simulink model "hybrid_new_eq_circuit_pascal5_single_shot_stack"  (R2019a)
settings: Solver=FixedStepAuto  StartTime=0.0  StopTime=sim_time  FixedStep=resolution  MinStep=0.001  RelTol=1e-4  EnableMultiTasking=on
values from neighbouring files (symbols this model uses):
  amps_in = double(amps_in)    [Sc.m]    (also in sc_model_single_shot_stack.m; test.m = 0; workspace_nedc_basic_sc.mat = 0; workspace_test_model.mat = 0)
  batt_c = [0.25 0.25 0.25 0.25 0.25 0.25 0.25]    [workspace_test_model.mat]
  batt_r = [1 1 1 1 1 1 1 1]    [workspace_test_model.mat]
  resolution = double(resolution)    [Sc.m]    (also in sc_model_single_shot.m = 0.1; sc_model_single_shot_stack.m = 0.1; workspace_test_model.mat = 10)
  tStep = resolution    (= 0.1)    [Sc.m]    (also in testHyb.m = 10; workspace_test_model.mat = 10)
undefined symbols (not defined in the file or in its folder): cCap, cR
libraries: powerlib x525, simulink x9
(part 2 of 8)

== system hybrid_new_eq_circuit_pascal5_single_shot_stack/Supercapacitor 2 ==
  note: 1x 4k
  note: 1x 550R
  note: 4x 625R
  note: 4x 1k4
  note: 6x 700R
  Bus Creator : BusCreator  Inputs=11
  Subsystem : Subsystem  mask{c=c(2), r_esr=r(2), r_leak=r_leak, v_init=v_init2}
      mask prompts: c "Capacitance /F"; r_esr "Series resistance /ohm"; r_leak "Leak resistance /ohm (inf for disabled)"; v_init "Initial capacitor voltage"
  Subsystem1 : Subsystem  mask{c=c(4), r_esr=r(4), r_leak=r_leak, v_init=v_init4}
      mask prompts: c "Capacitance /F"; r_esr "Series resistance /ohm"; r_leak "Leak resistance /ohm (inf for disabled)"; v_init "Initial capacitor voltage"
  Subsystem2 : Subsystem  mask{c=c(3), r_esr=r(3), r_leak=r_leak, v_init=v_init3}
      mask prompts: c "Capacitance /F"; r_esr "Series resistance /ohm"; r_leak "Leak resistance /ohm (inf for disabled)"; v_init "Initial capacitor voltage"
  Subsystem5 : Subsystem  mask{c=c(5), r_esr=r(5), r_leak=r_leak, v_init=v_init5}
      mask prompts: c "Capacitance /F"; r_esr "Series resistance /ohm"; r_leak "Leakage resistance /ohm (inf for disabled)"; v_init "Initial capacitor voltage"
  Subsystem8 : Subsystem  mask{c=c(1), r_esr=r(1), r_leak=r_leak, v_init=v_init1}
      mask prompts: c "Capacitance /F"; r_esr "Series resistance /ohm"; r_leak "Leakage resistance /ohm (inf for disabled)"; v_init "Initial capacitor voltage"
  v_cap_single : powerlib/Measurements/Voltage Measurement  PhasorSimulation=off  OutputType=Complex  PSBequivalent=0
      settings: SourceProductName=Simscape Electrical
  VCC_in : PMIOPort  Side=Left
  VSS_in : PMIOPort  Port=2  Side=Left
  VCC_out : PMIOPort  Port=3  Side=Right
  VSS_out : PMIOPort  Port=4  Side=Right
  v_r_out : Outport
  v_cap_out : Outport  Port=2
  i_leak_out : Outport  Port=3
  p_chg_out : Outport  Port=4
  p_leak_out : Outport  Port=5
  i_out : Outport  Port=6
  c_out : Outport  Port=7
  r_out : Outport  Port=8
  r_leak_out : Outport  Port=9
  bus_out : Outport  Port=10
  wires:
  Bus Creator/1 -> bus_out/1
  Subsystem5/10(l_out) -> Bus Creator/10
  v_cap_single/1 -> Bus Creator/11
  Subsystem2/7(Out7) -> Subsystem1/7(In7)
  Subsystem2/4(Out4) -> Subsystem1/4(In4)
  Subsystem2/3(Out3) -> Subsystem1/3(In3)
  Subsystem2/1(Out1) -> Subsystem1/1(In1)
  Subsystem2/9(Out9) -> Subsystem1/9(In9)
  Subsystem2/10(Out10) -> Subsystem1/10(In10)
  Subsystem2/2(Out2) -> Subsystem1/2(In2)
  Subsystem2/6(Out6) -> Subsystem1/6(In6)
  Subsystem2/8(Out8) -> Subsystem1/8(In8)
  Subsystem2/5(Out5) -> Subsystem1/5(In5)
  Subsystem/5(Out5) -> Subsystem2/5(In5)
  Subsystem/4(Out4) -> Subsystem2/4(In4)
  Subsystem/7(Out7) -> Subsystem2/7(In7)
  Subsystem/9(Out9) -> Subsystem2/9(In9)
  Subsystem/6(Out6) -> Subsystem2/6(In6)
  Subsystem/2(Out2) -> Subsystem2/2(In2)
  Subsystem/1(Out1) -> Subsystem2/1(In1)
  Subsystem/8(Out8) -> Subsystem2/8(In8)
  Subsystem/10(Out10) -> Subsystem2/10(In10)
  Subsystem/3(Out3) -> Subsystem2/3(In3)
  Subsystem1/1(Out1) -> Subsystem5/1(v_r_in)
  Subsystem1/2(Out2) -> Subsystem5/2(v_cap_in)
  Subsystem1/5(Out5) -> Subsystem5/5(p_leak_in)
  Subsystem1/10(Out10) -> Subsystem5/10(l_in)
  Subsystem1/3(Out3) -> Subsystem5/3(i_leak_in)
  Subsystem1/9(Out9) -> Subsystem5/9(r_leak_in)
  Subsystem1/7(Out7) -> Subsystem5/7(c_in)
  Subsystem1/4(Out4) -> Subsystem5/4(p_chg_in)
  Subsystem1/8(Out8) -> Subsystem5/8(r_in)
  Subsystem1/6(Out6) -> Subsystem5/6(i_in)
  Subsystem8/2(v_cap_out) -> Subsystem/2(In2)
  Subsystem8/1(v_r_out) -> Subsystem/1(In1)
  Subsystem8/7(c_out) -> Subsystem/7(In7)
  Subsystem8/5(p_leak_out) -> Subsystem/5(In5)
  Subsystem8/8(r_out) -> Subsystem/8(In8)
  Subsystem8/10(l_out) -> Subsystem/10(In10)
  Subsystem8/4(p_chg_out) -> Subsystem/4(In4)
  Subsystem8/9(r_leak_out) -> Subsystem/9(In9)
  Subsystem8/6(i_out) -> Subsystem/6(In6)
  Subsystem8/3(i_leak_out) -> Subsystem/3(In3)
  Subsystem5/1(v_r_out) -> v_r_out/1, Bus Creator/1
  Subsystem5/9(r_leak_out) -> r_leak_out/1, Bus Creator/9
  Subsystem5/2(v_cap_out) -> v_cap_out/1, Bus Creator/2
  Subsystem5/8(r_out) -> r_out/1, Bus Creator/8
  Subsystem5/3(i_leak_out) -> i_leak_out/1, Bus Creator/3
  Subsystem5/7(c_out) -> c_out/1, Bus Creator/7
  Subsystem5/4(p_chg_out) -> p_chg_out/1, Bus Creator/4
  Subsystem5/6(i_out) -> i_out/1, Bus Creator/6
  Subsystem5/5(p_leak_out) -> p_leak_out/1, Bus Creator/5
  connections:
  VSS_out/RConn1 -- v_cap_single/LConn2 -- Subsystem5/RConn2
  Subsystem5/RConn1 -- v_cap_single/LConn1 -- VCC_out/RConn1
  Subsystem1/LConn1 -- Subsystem2/RConn1
  Subsystem1/LConn2 -- Subsystem2/RConn2
  Subsystem/RConn2 -- Subsystem2/LConn2
  Subsystem/RConn1 -- Subsystem2/LConn1
  Subsystem1/RConn1 -- Subsystem5/LConn1
  Subsystem1/RConn2 -- Subsystem5/LConn2
  Subsystem8/RConn1 -- Subsystem/LConn1
  Subsystem8/RConn2 -- Subsystem/LConn2
  VSS_in/RConn1 -- Subsystem8/LConn2
  Subsystem8/LConn1 -- VCC_in/RConn1

== system hybrid_new_eq_circuit_pascal5_single_shot_stack/Supercapacitor 3 ==
  note: 6x 700R
  note: 4x 1k4
  note: 4x 625R
  note: 1x 550R
  note: 1x 4k
  Bus Creator : BusCreator  Inputs=11
  Subsystem : Subsystem  mask{c=c(2), r_esr=r(2), r_leak=r_leak, v_init=v_init2}
      mask prompts: c "Capacitance /F"; r_esr "Series resistance /ohm"; r_leak "Leak resistance /ohm (inf for disabled)"; v_init "Initial capacitor voltage"
  Subsystem1 : Subsystem  mask{c=c(4), r_esr=r(4), r_leak=r_leak, v_init=v_init4}
      mask prompts: c "Capacitance /F"; r_esr "Series resistance /ohm"; r_leak "Leak resistance /ohm (inf for disabled)"; v_init "Initial capacitor voltage"
  Subsystem2 : Subsystem  mask{c=c(3), r_esr=r(3), r_leak=r_leak, v_init=v_init3}
      mask prompts: c "Capacitance /F"; r_esr "Series resistance /ohm"; r_leak "Leak resistance /ohm (inf for disabled)"; v_init "Initial capacitor voltage"
  Subsystem5 : Subsystem  mask{c=c(5), r_esr=r(5), r_leak=r_leak, v_init=v_init5}
      mask prompts: c "Capacitance /F"; r_esr "Series resistance /ohm"; r_leak "Leakage resistance /ohm (inf for disabled)"; v_init "Initial capacitor voltage"
  Subsystem8 : Subsystem  mask{c=c(1), r_esr=r(1), r_leak=r_leak, v_init=v_init1}
      mask prompts: c "Capacitance /F"; r_esr "Series resistance /ohm"; r_leak "Leakage resistance /ohm (inf for disabled)"; v_init "Initial capacitor voltage"
  v_cap_single : powerlib/Measurements/Voltage Measurement  PhasorSimulation=off  OutputType=Complex  PSBequivalent=0
      settings: SourceProductName=Simscape Electrical
  VCC_in : PMIOPort  Side=Left
  VSS_in : PMIOPort  Port=2  Side=Left
  VCC_out : PMIOPort  Port=3  Side=Right
  VSS_out : PMIOPort  Port=4  Side=Right
  v_r_out : Outport
  v_cap_out : Outport  Port=2
  i_leak_out : Outport  Port=3
  p_chg_out : Outport  Port=4
  p_leak_out : Outport  Port=5
  i_out : Outport  Port=6
  c_out : Outport  Port=7
  r_out : Outport  Port=8
  r_leak_out : Outport  Port=9
  bus_out : Outport  Port=10
  wires:
  Subsystem5/5(p_leak_out) -> Bus Creator/5, p_leak_out/1
  Subsystem5/6(i_out) -> Bus Creator/6, i_out/1
  Subsystem5/4(p_chg_out) -> Bus Creator/4, p_chg_out/1
  Subsystem5/7(c_out) -> Bus Creator/7, c_out/1
  Subsystem5/3(i_leak_out) -> Bus Creator/3, i_leak_out/1
  Subsystem5/8(r_out) -> Bus Creator/8, r_out/1
  Subsystem5/2(v_cap_out) -> Bus Creator/2, v_cap_out/1
  Subsystem5/9(r_leak_out) -> Bus Creator/9, r_leak_out/1
  Subsystem5/1(v_r_out) -> Bus Creator/1, v_r_out/1
  Subsystem8/3(i_leak_out) -> Subsystem/3(In3)
  Subsystem8/6(i_out) -> Subsystem/6(In6)
  Subsystem8/9(r_leak_out) -> Subsystem/9(In9)
  Subsystem8/4(p_chg_out) -> Subsystem/4(In4)
  Subsystem8/10(l_out) -> Subsystem/10(In10)
  Subsystem8/8(r_out) -> Subsystem/8(In8)
  Subsystem8/5(p_leak_out) -> Subsystem/5(In5)
  Subsystem8/7(c_out) -> Subsystem/7(In7)
  Subsystem8/1(v_r_out) -> Subsystem/1(In1)
  Subsystem8/2(v_cap_out) -> Subsystem/2(In2)
  Subsystem1/6(Out6) -> Subsystem5/6(i_in)
  Subsystem1/8(Out8) -> Subsystem5/8(r_in)
  Subsystem1/4(Out4) -> Subsystem5/4(p_chg_in)
  Subsystem1/7(Out7) -> Subsystem5/7(c_in)
  Subsystem1/9(Out9) -> Subsystem5/9(r_leak_in)
  Subsystem1/3(Out3) -> Subsystem5/3(i_leak_in)
  Subsystem1/10(Out10) -> Subsystem5/10(l_in)
  Subsystem1/5(Out5) -> Subsystem5/5(p_leak_in)
  Subsystem1/2(Out2) -> Subsystem5/2(v_cap_in)
  Subsystem1/1(Out1) -> Subsystem5/1(v_r_in)
  Subsystem/3(Out3) -> Subsystem2/3(In3)
  Subsystem/10(Out10) -> Subsystem2/10(In10)
  Subsystem/8(Out8) -> Subsystem2/8(In8)
  Subsystem/1(Out1) -> Subsystem2/1(In1)
  Subsystem/2(Out2) -> Subsystem2/2(In2)
  Subsystem/6(Out6) -> Subsystem2/6(In6)
  Subsystem/9(Out9) -> Subsystem2/9(In9)
  Subsystem/7(Out7) -> Subsystem2/7(In7)
  Subsystem/4(Out4) -> Subsystem2/4(In4)
  Subsystem/5(Out5) -> Subsystem2/5(In5)
  Subsystem2/5(Out5) -> Subsystem1/5(In5)
  Subsystem2/8(Out8) -> Subsystem1/8(In8)
  Subsystem2/6(Out6) -> Subsystem1/6(In6)
  Subsystem2/2(Out2) -> Subsystem1/2(In2)
  Subsystem2/10(Out10) -> Subsystem1/10(In10)
  Subsystem2/9(Out9) -> Subsystem1/9(In9)
  Subsystem2/1(Out1) -> Subsystem1/1(In1)
  Subsystem2/3(Out3) -> Subsystem1/3(In3)
  Subsystem2/4(Out4) -> Subsystem1/4(In4)
  Subsystem2/7(Out7) -> Subsystem1/7(In7)
  v_cap_single/1 -> Bus Creator/11
  Subsystem5/10(l_out) -> Bus Creator/10
  Bus Creator/1 -> bus_out/1
  connections:
  Subsystem8/LConn1 -- VCC_in/RConn1
  VSS_in/RConn1 -- Subsystem8/LConn2
  Subsystem8/RConn2 -- Subsystem/LConn2
  Subsystem8/RConn1 -- Subsystem/LConn1
  Subsystem1/RConn2 -- Subsystem5/LConn2
  Subsystem1/RConn1 -- Subsystem5/LConn1
  Subsystem/RConn1 -- Subsystem2/LConn1
  Subsystem/RConn2 -- Subsystem2/LConn2
  Subsystem1/LConn2 -- Subsystem2/RConn2
  Subsystem1/LConn1 -- Subsystem2/RConn1
  VCC_out/RConn1 -- v_cap_single/LConn1 -- Subsystem5/RConn1
  Subsystem5/RConn2 -- v_cap_single/LConn2 -- VSS_out/RConn1

== system hybrid_new_eq_circuit_pascal5_single_shot_stack/Battery 1/Subsystem ==
  In1 : Inport
  In2 : Inport  Port=2
  In3 : Inport  Port=3
  In4 : Inport  Port=4
  In5 : Inport  Port=5
  In6 : Inport  Port=6
  In7 : Inport  Port=7
  In8 : Inport  Port=8
  In9 : Inport  Port=9
  In10 : Inport  Port=10
  Subsystem1 : Subsystem  mask{c=c(5), r_esr=r(5), r_leak=r_leak, v_init=v_init(5)}
      mask prompts: c "Capacitance /F"; r_esr "Series resistance /ohm"; r_leak "Leakage resistance /ohm (inf for disabled)"; v_init "Initial capacitor voltage"
  Subsystem2 : Subsystem  mask{c=c(6), r_esr=r(6), r_leak=r_leak, v_init=v_init(6)}
      mask prompts: c "Capacitance /F"; r_esr "Series resistance /ohm"; r_leak "Leakage resistance /ohm (inf for disabled)"; v_init "Initial capacitor voltage"
  Subsystem3 : Subsystem  mask{c=c(7), r_esr=r(7), r_leak=r_leak, v_init=v_init(7)}
      mask prompts: c "Capacitance /F"; r_esr "Series resistance /ohm"; r_leak "Leakage resistance /ohm (inf for disabled)"; v_init "Initial capacitor voltage"
  Subsystem5 : Subsystem  mask{c=c(4), r_esr=r(4), r_leak=r_leak, v_init=v_init(4)}
      mask prompts: c "Capacitance /F"; r_esr "Series resistance /ohm"; r_leak "Leakage resistance /ohm (inf for disabled)"; v_init "Initial capacitor voltage"
  VCC_in : PMIOPort  Side=Left
  VCC_out : PMIOPort  Port=2  Side=Right
  VSS_in : PMIOPort  Port=3  Side=Left
  VSS_out : PMIOPort  Port=4  Side=Right
  Out1 : Outport
  Out2 : Outport  Port=2
  Out3 : Outport  Port=3
  Out4 : Outport  Port=4
  Out5 : Outport  Port=5
  Out6 : Outport  Port=6
  Out7 : Outport  Port=7
  Out8 : Outport  Port=8
  Out9 : Outport  Port=9
  Out10 : Outport  Port=10
  wires:
  In2/1 -> Subsystem5/2(v_cap_in)
  In9/1 -> Subsystem5/9(r_leak_in)
  In6/1 -> Subsystem5/6(i_in)
  In5/1 -> Subsystem5/5(p_leak_in)
  In4/1 -> Subsystem5/4(p_chg_in)
  In7/1 -> Subsystem5/7(c_in)
  In1/1 -> Subsystem5/1(v_r_in)
  In10/1 -> Subsystem5/10(l_in)
  In3/1 -> Subsystem5/3(i_leak_in)
  In8/1 -> Subsystem5/8(r_in)
  Subsystem5/1(v_r_out) -> Subsystem1/1(v_r_in)
  Subsystem5/2(v_cap_out) -> Subsystem1/2(v_cap_in)
  Subsystem5/3(i_leak_out) -> Subsystem1/3(i_leak_in)
  Subsystem5/4(p_chg_out) -> Subsystem1/4(p_chg_in)
  Subsystem5/5(p_leak_out) -> Subsystem1/5(p_leak_in)
  Subsystem5/6(i_out) -> Subsystem1/6(i_in)
  Subsystem5/7(c_out) -> Subsystem1/7(c_in)
  Subsystem5/8(r_out) -> Subsystem1/8(r_in)
  Subsystem5/9(r_leak_out) -> Subsystem1/9(r_leak_in)
  Subsystem5/10(l_out) -> Subsystem1/10(l_in)
  Subsystem1/1(v_r_out) -> Subsystem2/1(v_r_in)
  Subsystem1/2(v_cap_out) -> Subsystem2/2(v_cap_in)
  Subsystem1/3(i_leak_out) -> Subsystem2/3(i_leak_in)
  Subsystem1/4(p_chg_out) -> Subsystem2/4(p_chg_in)
  Subsystem1/5(p_leak_out) -> Subsystem2/5(p_leak_in)
  Subsystem1/6(i_out) -> Subsystem2/6(i_in)
  Subsystem1/7(c_out) -> Subsystem2/7(c_in)
  Subsystem1/8(r_out) -> Subsystem2/8(r_in)
  Subsystem1/9(r_leak_out) -> Subsystem2/9(r_leak_in)
  Subsystem1/10(l_out) -> Subsystem2/10(l_in)
  Subsystem2/1(v_r_out) -> Subsystem3/1(v_r_in)
  Subsystem2/2(v_cap_out) -> Subsystem3/2(v_cap_in)
  Subsystem2/3(i_leak_out) -> Subsystem3/3(i_leak_in)
  Subsystem2/4(p_chg_out) -> Subsystem3/4(p_chg_in)
  Subsystem2/5(p_leak_out) -> Subsystem3/5(p_leak_in)
  Subsystem2/6(i_out) -> Subsystem3/6(i_in)
  Subsystem2/7(c_out) -> Subsystem3/7(c_in)
  Subsystem2/8(r_out) -> Subsystem3/8(r_in)
  Subsystem2/9(r_leak_out) -> Subsystem3/9(r_leak_in)
  Subsystem2/10(l_out) -> Subsystem3/10(l_in)
  Subsystem3/1(v_r_out) -> Out1/1
  Subsystem3/2(v_cap_out) -> Out2/1
  Subsystem3/3(i_leak_out) -> Out3/1
  Subsystem3/4(p_chg_out) -> Out4/1
  Subsystem3/5(p_leak_out) -> Out5/1
  Subsystem3/6(i_out) -> Out6/1
  Subsystem3/7(c_out) -> Out7/1
  Subsystem3/8(r_out) -> Out8/1
  Subsystem3/9(r_leak_out) -> Out9/1
  Subsystem3/10(l_out) -> Out10/1
  connections:
  Subsystem5/LConn1 -- VCC_in/RConn1
  Subsystem5/LConn2 -- VSS_in/RConn1
  Subsystem5/RConn1 -- Subsystem1/LConn1
  Subsystem5/RConn2 -- Subsystem1/LConn2
  Subsystem1/RConn1 -- Subsystem2/LConn1
  Subsystem1/RConn2 -- Subsystem2/LConn2
  Subsystem2/RConn1 -- Subsystem3/LConn1
  Subsystem2/RConn2 -- Subsystem3/LConn2
  Subsystem3/RConn1 -- VCC_out/RConn1
  Subsystem3/RConn2 -- VSS_out/RConn1

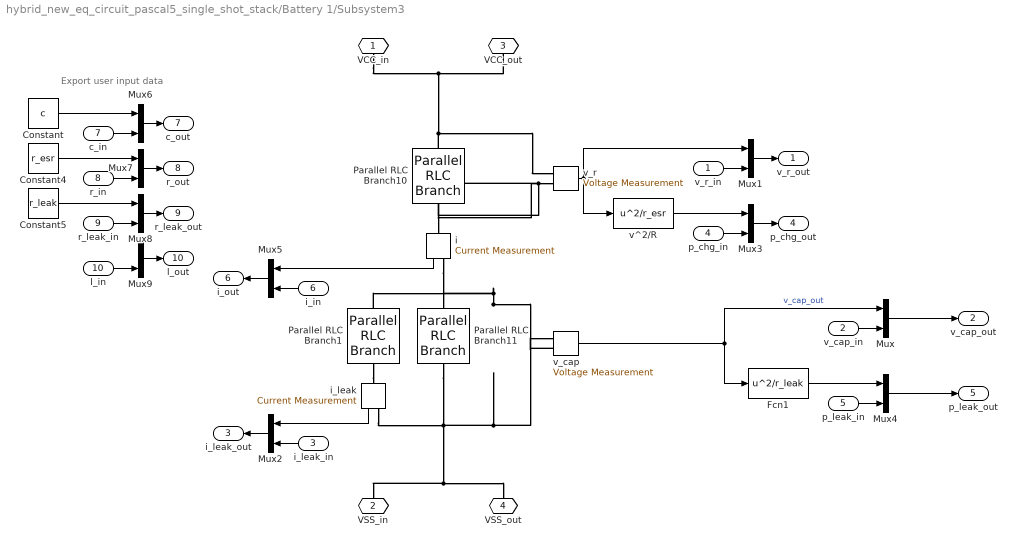
== system hybrid_new_eq_circuit_pascal5_single_shot_stack/Battery 1/Subsystem3 ==
  note: Export user input data
  v_r_in : Inport
  v_cap_in : Inport  Port=2
  i_leak_in : Inport  Port=3
  p_chg_in : Inport  Port=4
  p_leak_in : Inport  Port=5
  i_in : Inport  Port=6
  c_in : Inport  Port=7
  r_in : Inport  Port=8
  r_leak_in : Inport  Port=9
  l_in : Inport  Port=10
  Constant : Constant  Value=c
  Constant4 : Constant  Value=r_esr
  Constant5 : Constant  Value=r_leak
  Fcn1 : Fcn  Expr=u^2/r_leak
  Mux{,1..9} (10 alike) : Mux  Inputs=2
  Parallel RLC Branch1 : powerlib/Elements/Parallel RLC Branch  LConnTagsString=a  RConnTagsString=__new0  BranchType=R  Resistance=r_esr  Inductance=1e-3  SetiL0=off  InitialCurrent=0  Capacitance=1e-6  Setx0=off  InitialVoltage=0  Measurements=None
      settings: SourceProductName=Simscape Electrical
  Parallel RLC Branch10 : powerlib/Elements/Parallel RLC Branch  LConnTagsString=a  RConnTagsString=__new0  BranchType=R  Resistance=0.000001  Inductance=1e-3  SetiL0=off  InitialCurrent=0  Capacitance=1e-6  Setx0=off  InitialVoltage=0  Measurements=None
      settings: SourceProductName=Simscape Electrical
  Parallel RLC Branch11 : powerlib/Elements/Parallel RLC Branch  LConnTagsString=a  RConnTagsString=__new0  BranchType=C  Resistance=1  Inductance=1e-3  SetiL0=off  InitialCurrent=0  Capacitance=c  Setx0=on  InitialVoltage=v_init  Measurements=None
      settings: SourceProductName=Simscape Electrical
  i : powerlib/Measurements/Current Measurement  PhasorSimulation=off  OutputType=Complex  PSBequivalent=0
      settings: SourceProductName=Simscape Electrical
  i_leak : powerlib/Measurements/Current Measurement  PhasorSimulation=off  OutputType=Complex  PSBequivalent=0
      settings: SourceProductName=Simscape Electrical
  v^2/R : Fcn  Expr=u^2/r_esr
  v_cap : powerlib/Measurements/Voltage Measurement  PhasorSimulation=off  OutputType=Magnitude  PSBequivalent=0
      settings: SourceProductName=Simscape Electrical
  v_r : powerlib/Measurements/Voltage Measurement  PhasorSimulation=off  OutputType=Complex  PSBequivalent=0
      settings: SourceProductName=Simscape Electrical
  VCC_in : PMIOPort  Side=Left
  VSS_in : PMIOPort  Port=2  Side=Left
  VCC_out : PMIOPort  Tag=PMCPort  Port=3  Side=Right
  VSS_out : PMIOPort  Tag=PMCPort  Port=4  Side=Right
  v_r_out : Outport
  v_cap_out : Outport  Port=2
  i_leak_out : Outport  Port=3
  p_chg_out : Outport  Port=4
  p_leak_out : Outport  Port=5
  i_out : Outport  Port=6
  c_out : Outport  Port=7
  r_out : Outport  Port=8
  r_leak_out : Outport  Port=9
  l_out : Outport  Port=10
  wires:
  i_leak/1 -> Mux2/1
  v_r/1 -> Mux1/1, v^2/R/1
  Mux6/1 -> c_out/1
  Mux7/1 -> r_out/1
  Mux8/1 -> r_leak_out/1
  Mux9/1 -> l_out/1
  Constant/1 -> Mux6/1
  Constant4/1 -> Mux7/1
  Constant5/1 -> Mux8/1
  ? -> Mux9/1
  c_in/1 -> Mux6/2
  l_in/1 -> Mux9/2
  r_leak_in/1 -> Mux8/2
  r_in/1 -> Mux7/2
  p_chg_in/1 -> Mux3/2
  Mux3/1 -> p_chg_out/1
  v_r_in/1 -> Mux1/2
  Mux1/1 -> v_r_out/1
  v^2/R/1 -> Mux3/1
  Mux2/1 -> i_leak_out/1
  i_leak_in/1 -> Mux2/2
  i/1 -> Mux5/1
  Mux5/1 -> i_out/1
  i_in/1 -> Mux5/2
  p_leak_in/1 -> Mux4/2
  Mux4/1 -> p_leak_out/1
  Mux/1 -> v_cap_out/1
  v_cap_in/1 -> Mux/2
  Fcn1/1 -> Mux4/1
  v_cap/1 -> Fcn1/1, Mux/1  "v_cap_out"
  connections:
  VCC_in/RConn1 -- VCC_out/RConn1 -- v_r/LConn1 -- Parallel RLC Branch10/LConn1
  Parallel RLC Branch1/RConn1 -- i_leak/LConn1
  VSS_out/RConn1 -- VSS_in/RConn1 -- i_leak/RConn1 -- Parallel RLC Branch11/RConn1 -- v_cap/LConn2
  Parallel RLC Branch1/LConn1 -- i/RConn1 -- Parallel RLC Branch11/LConn1 -- v_cap/LConn1
  v_r/LConn2 -- Parallel RLC Branch10/RConn1 -- i/LConn1

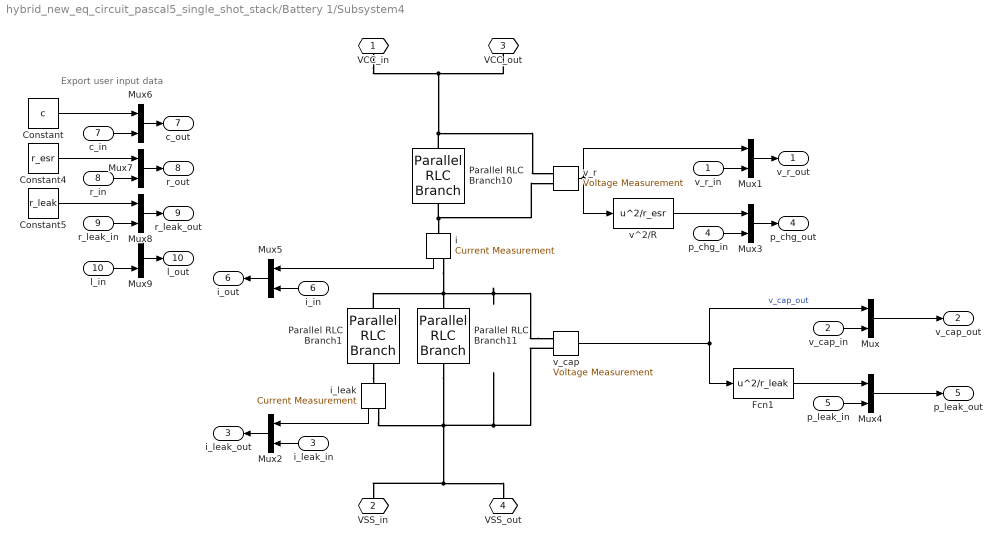
== system hybrid_new_eq_circuit_pascal5_single_shot_stack/Battery 1/Subsystem4 ==
  note: Export user input data
  v_r_in : Inport
  v_cap_in : Inport  Port=2
  i_leak_in : Inport  Port=3
  p_chg_in : Inport  Port=4
  p_leak_in : Inport  Port=5
  i_in : Inport  Port=6
  c_in : Inport  Port=7
  r_in : Inport  Port=8
  r_leak_in : Inport  Port=9
  l_in : Inport  Port=10
  Constant : Constant  Value=c
  Constant4 : Constant  Value=r_esr
  Constant5 : Constant  Value=r_leak
  Fcn1 : Fcn  Expr=u^2/r_leak
  Mux{,1..9} (10 alike) : Mux  Inputs=2
  Parallel RLC Branch1 : powerlib/Elements/Parallel RLC Branch  LConnTagsString=a  RConnTagsString=__new0  BranchType=R  Resistance=r_esr  Inductance=1e-3  SetiL0=off  InitialCurrent=0  Capacitance=1e-6  Setx0=off  InitialVoltage=0  Measurements=None
      settings: SourceProductName=Simscape Electrical
  Parallel RLC Branch10 : powerlib/Elements/Parallel RLC Branch  LConnTagsString=a  RConnTagsString=__new0  BranchType=R  Resistance=0.000001  Inductance=1e-3  SetiL0=off  InitialCurrent=0  Capacitance=1e-6  Setx0=off  InitialVoltage=0  Measurements=None
      settings: SourceProductName=Simscape Electrical
  Parallel RLC Branch11 : powerlib/Elements/Parallel RLC Branch  LConnTagsString=a  RConnTagsString=__new0  BranchType=C  Resistance=1  Inductance=1e-3  SetiL0=off  InitialCurrent=0  Capacitance=c  Setx0=on  InitialVoltage=v_init  Measurements=None
      settings: SourceProductName=Simscape Electrical
  i : powerlib/Measurements/Current Measurement  PhasorSimulation=off  OutputType=Complex  PSBequivalent=0
      settings: SourceProductName=Simscape Electrical
  i_leak : powerlib/Measurements/Current Measurement  PhasorSimulation=off  OutputType=Complex  PSBequivalent=0
      settings: SourceProductName=Simscape Electrical
  v^2/R : Fcn  Expr=u^2/r_esr
  v_cap : powerlib/Measurements/Voltage Measurement  PhasorSimulation=off  OutputType=Magnitude  PSBequivalent=0
      settings: SourceProductName=Simscape Electrical
  v_r : powerlib/Measurements/Voltage Measurement  PhasorSimulation=off  OutputType=Complex  PSBequivalent=0
      settings: SourceProductName=Simscape Electrical
  VCC_in : PMIOPort  Side=Left
  VSS_in : PMIOPort  Port=2  Side=Left
  VCC_out : PMIOPort  Tag=PMCPort  Port=3  Side=Right
  VSS_out : PMIOPort  Tag=PMCPort  Port=4  Side=Right
  v_r_out : Outport
  v_cap_out : Outport  Port=2
  i_leak_out : Outport  Port=3
  p_chg_out : Outport  Port=4
  p_leak_out : Outport  Port=5
  i_out : Outport  Port=6
  c_out : Outport  Port=7
  r_out : Outport  Port=8
  r_leak_out : Outport  Port=9
  l_out : Outport  Port=10
  wires:
  Fcn1/1 -> Mux4/1
  v_cap_in/1 -> Mux/2
  Mux/1 -> v_cap_out/1
  Mux4/1 -> p_leak_out/1
  p_leak_in/1 -> Mux4/2
  i_in/1 -> Mux5/2
  Mux5/1 -> i_out/1
  i/1 -> Mux5/1
  i_leak_in/1 -> Mux2/2
  Mux2/1 -> i_leak_out/1
  v^2/R/1 -> Mux3/1
  Mux1/1 -> v_r_out/1
  v_r_in/1 -> Mux1/2
  Mux3/1 -> p_chg_out/1
  p_chg_in/1 -> Mux3/2
  r_in/1 -> Mux7/2
  r_leak_in/1 -> Mux8/2
  l_in/1 -> Mux9/2
  c_in/1 -> Mux6/2
  ? -> Mux9/1
  Constant5/1 -> Mux8/1
  Constant4/1 -> Mux7/1
  Constant/1 -> Mux6/1
  Mux9/1 -> l_out/1
  Mux8/1 -> r_leak_out/1
  Mux7/1 -> r_out/1
  Mux6/1 -> c_out/1
  v_r/1 -> v^2/R/1, Mux1/1
  i_leak/1 -> Mux2/1
  v_cap/1 -> Mux/1, Fcn1/1  "v_cap_out"
  connections:
  i/LConn1 -- Parallel RLC Branch10/RConn1 -- v_r/LConn2
  Parallel RLC Branch10/LConn1 -- VCC_in/RConn1 -- VCC_out/RConn1 -- v_r/LConn1
  v_cap/LConn1 -- Parallel RLC Branch11/LConn1 -- i/RConn1 -- Parallel RLC Branch1/LConn1
  v_cap/LConn2 -- Parallel RLC Branch11/RConn1 -- i_leak/RConn1 -- VSS_in/RConn1 -- VSS_out/RConn1
  Parallel RLC Branch1/RConn1 -- i_leak/LConn1

== system hybrid_new_eq_circuit_pascal5_single_shot_stack/Battery 1/Subsystem8 ==
  note: Export user input data
  Constant : Constant  Value=c
  Constant4 : Constant  Value=r_esr
  Constant5 : Constant  Value=r_leak
  Fcn1 : Fcn  Expr=u^2/r_leak
  Parallel RLC Branch1 : powerlib/Elements/Parallel RLC Branch  LConnTagsString=a  RConnTagsString=__new0  BranchType=R  Resistance=r_leak  Inductance=1e-3  SetiL0=off  InitialCurrent=0  Capacitance=1e-6  Setx0=off  InitialVoltage=0  Measurements=None
      settings: SourceProductName=Simscape Electrical
  Parallel RLC Branch10 : powerlib/Elements/Parallel RLC Branch  LConnTagsString=a  RConnTagsString=__new0  BranchType=R  Resistance=0.000001  Inductance=1e-3  SetiL0=off  InitialCurrent=0  Capacitance=1e-6  Setx0=off  InitialVoltage=0  Measurements=None
      settings: SourceProductName=Simscape Electrical
  Parallel RLC Branch11 : powerlib/Elements/Parallel RLC Branch  LConnTagsString=a  RConnTagsString=__new0  BranchType=C  Resistance=1  Inductance=1e-3  SetiL0=off  InitialCurrent=0  Capacitance=c  Setx0=on  InitialVoltage=v_init  Measurements=None
      settings: SourceProductName=Simscape Electrical
  i : powerlib/Measurements/Current Measurement  PhasorSimulation=off  OutputType=Complex  PSBequivalent=0
      settings: SourceProductName=Simscape Electrical
  i_leak : powerlib/Measurements/Current Measurement  PhasorSimulation=off  OutputType=Complex  PSBequivalent=0
      settings: SourceProductName=Simscape Electrical
  v^2/R : Fcn  Expr=u^2/r_esr
  v_cap : powerlib/Measurements/Voltage Measurement  PhasorSimulation=off  OutputType=Magnitude  PSBequivalent=0
      settings: SourceProductName=Simscape Electrical
  v_r : powerlib/Measurements/Voltage Measurement  PhasorSimulation=off  OutputType=Complex  PSBequivalent=0
      settings: SourceProductName=Simscape Electrical
  VCC_in : PMIOPort  Side=Left
  VSS_in : PMIOPort  Port=2  Side=Left
  VCC_out : PMIOPort  Tag=PMCPort  Port=3  Side=Right
  VSS_out : PMIOPort  Tag=PMCPort  Port=4  Side=Right
  v_r_out : Outport
  v_cap_out : Outport  Port=2
  i_leak_out : Outport  Port=3
  p_chg_out : Outport  Port=4
  p_leak_out : Outport  Port=5
  i_out : Outport  Port=6
  c_out : Outport  Port=7
  r_out : Outport  Port=8
  r_leak_out : Outport  Port=9
  l_out : Outport  Port=10
  wires:
  v^2/R/1 -> p_chg_out/1
  Fcn1/1 -> p_leak_out/1
  v_cap/1 -> Fcn1/1, v_cap_out/1  "v_cap_out"
  i/1 -> i_out/1
  ? -> l_out/1
  Constant5/1 -> r_leak_out/1
  Constant4/1 -> r_out/1
  Constant/1 -> c_out/1
  v_r/1 -> v^2/R/1, v_r_out/1
  i_leak/1 -> i_leak_out/1
  connections:
  v_r/LConn2 -- Parallel RLC Branch10/RConn1 -- i/LConn1
  Parallel RLC Branch1/RConn1 -- i_leak/LConn1
  Parallel RLC Branch10/LConn1 -- v_r/LConn1 -- VCC_out/RConn1 -- VCC_in/RConn1
  v_cap/LConn1 -- i/RConn1 -- Parallel RLC Branch1/LConn1 -- Parallel RLC Branch11/LConn1
  VSS_in/RConn1 -- VSS_out/RConn1 -- i_leak/RConn1 -- v_cap/LConn2 -- Parallel RLC Branch11/RConn1

== system hybrid_new_eq_circuit_pascal5_single_shot_stack/Battery 2/Bus Merge2 ==
  bus_1_in : Inport
  bus_2_in : Inport  Port=2
  Bus Creator : BusCreator  Inputs=11
  Bus Selector : BusSelector  OutputSignals=signal1,v_cap_out,signal3,signal4,signal5,signal6,signal7,signal8,signal9,signal10,signal11
  Bus Selector1 : BusSelector  OutputSignals=signal1,v_cap_out,signal3,signal4,signal5,signal6,signal7,signal8,signal9,signal10,signal11
  Mux{1..11} (11 alike) : Mux  Inputs=2
  bus_out : Outport
  wires:
  bus_1_in/1 -> Bus Selector/1
  bus_2_in/1 -> Bus Selector1/1
  Bus Creator/1 -> bus_out/1
  Bus Selector/1 -> Mux1/1  "<signal1>"
  Bus Selector1/2 -> Mux2/2  "<v_cap_out>"
  Bus Selector/3 -> Mux3/1  "<signal3>"
  Bus Selector1/4 -> Mux4/2  "<signal4>"
  Bus Selector/5 -> Mux5/1  "<signal5>"
  Bus Selector1/6 -> Mux6/1  "<signal6>"
  Bus Selector/7 -> Mux7/1  "<signal7>"
  Bus Selector1/8 -> Mux8/1  "<signal8>"
  Bus Selector1/10 -> Mux10/1  "<signal10>"
  Bus Selector/11 -> Mux11/1  "<signal11>"
  Bus Selector/9 -> Mux9/1  "<signal9>"
  Bus Selector/2 -> Mux2/1  "<v_cap_out>"
  Bus Selector/4 -> Mux4/1  "<signal4>"
  Bus Selector/6 -> Mux6/2  "<signal6>"
  Bus Selector/8 -> Mux8/2  "<signal8>"
  Bus Selector/10 -> Mux10/2  "<signal10>"
  Bus Selector1/1 -> Mux1/2  "<signal1>"
  Bus Selector1/3 -> Mux3/2  "<signal3>"
  Bus Selector1/5 -> Mux5/2  "<signal5>"
  Bus Selector1/7 -> Mux7/2  "<signal7>"
  Bus Selector1/9 -> Mux9/2  "<signal9>"
  Bus Selector1/11 -> Mux11/2  "<signal11>"
  Mux1/1 -> Bus Creator/1
  Mux3/1 -> Bus Creator/3
  Mux5/1 -> Bus Creator/5
  Mux7/1 -> Bus Creator/7
  Mux9/1 -> Bus Creator/9
  Mux11/1 -> Bus Creator/11
  Mux2/1 -> Bus Creator/2  "v_cap_out"
  Mux4/1 -> Bus Creator/4
  Mux6/1 -> Bus Creator/6
  Mux8/1 -> Bus Creator/8
  Mux10/1 -> Bus Creator/10

== system hybrid_new_eq_circuit_pascal5_single_shot_stack/Battery 2/Subsystem ==
  In1 : Inport
  In2 : Inport  Port=2
  In3 : Inport  Port=3
  In4 : Inport  Port=4
  In5 : Inport  Port=5
  In6 : Inport  Port=6
  In7 : Inport  Port=7
  In8 : Inport  Port=8
  In9 : Inport  Port=9
  In10 : Inport  Port=10
  Subsystem1 : Subsystem  mask{c=c(5), r_esr=r(5), r_leak=r_leak, v_init=v_init(5)}
      mask prompts: c "Capacitance /F"; r_esr "Series resistance /ohm"; r_leak "Leakage resistance /ohm (inf for disabled)"; v_init "Initial capacitor voltage"
  Subsystem2 : Subsystem  mask{c=c(6), r_esr=r(6), r_leak=r_leak, v_init=v_init(6)}
      mask prompts: c "Capacitance /F"; r_esr "Series resistance /ohm"; r_leak "Leakage resistance /ohm (inf for disabled)"; v_init "Initial capacitor voltage"
  Subsystem3 : Subsystem  mask{c=c(7), r_esr=r(7), r_leak=r_leak, v_init=v_init(7)}
      mask prompts: c "Capacitance /F"; r_esr "Series resistance /ohm"; r_leak "Leakage resistance /ohm (inf for disabled)"; v_init "Initial capacitor voltage"
  Subsystem5 : Subsystem  mask{c=c(4), r_esr=r(4), r_leak=r_leak, v_init=v_init(4)}
      mask prompts: c "Capacitance /F"; r_esr "Series resistance /ohm"; r_leak "Leakage resistance /ohm (inf for disabled)"; v_init "Initial capacitor voltage"
  Conn1 : PMIOPort  Side=Left
  Conn2 : PMIOPort  Port=2  Side=Right
  Conn3 : PMIOPort  Port=3  Side=Left
  Conn4 : PMIOPort  Port=4  Side=Right
  Out1 : Outport
  Out2 : Outport  Port=2
  Out3 : Outport  Port=3
  Out4 : Outport  Port=4
  Out5 : Outport  Port=5
  Out6 : Outport  Port=6
  Out7 : Outport  Port=7
  Out8 : Outport  Port=8
  Out9 : Outport  Port=9
  Out10 : Outport  Port=10
  wires:
  In2/1 -> Subsystem5/2(v_cap_in)
  In9/1 -> Subsystem5/9(r_leak_in)
  In6/1 -> Subsystem5/6(i_in)
  In5/1 -> Subsystem5/5(p_leak_in)
  In4/1 -> Subsystem5/4(p_chg_in)
  In7/1 -> Subsystem5/7(c_in)
  In1/1 -> Subsystem5/1(v_r_in)
  In10/1 -> Subsystem5/10(l_in)
  In3/1 -> Subsystem5/3(i_leak_in)
  In8/1 -> Subsystem5/8(r_in)
  Subsystem5/1(v_r_out) -> Subsystem1/1(v_r_in)
  Subsystem5/2(v_cap_out) -> Subsystem1/2(v_cap_in)
  Subsystem5/3(i_leak_out) -> Subsystem1/3(i_leak_in)
  Subsystem5/4(p_chg_out) -> Subsystem1/4(p_chg_in)
  Subsystem5/5(p_leak_out) -> Subsystem1/5(p_leak_in)
  Subsystem5/6(i_out) -> Subsystem1/6(i_in)
  Subsystem5/7(c_out) -> Subsystem1/7(c_in)
  Subsystem5/8(r_out) -> Subsystem1/8(r_in)
  Subsystem5/9(r_leak_out) -> Subsystem1/9(r_leak_in)
  Subsystem5/10(l_out) -> Subsystem1/10(l_in)
  Subsystem1/1(v_r_out) -> Subsystem2/1(v_r_in)
  Subsystem1/2(v_cap_out) -> Subsystem2/2(v_cap_in)
  Subsystem1/3(i_leak_out) -> Subsystem2/3(i_leak_in)
  Subsystem1/4(p_chg_out) -> Subsystem2/4(p_chg_in)
  Subsystem1/5(p_leak_out) -> Subsystem2/5(p_leak_in)
  Subsystem1/6(i_out) -> Subsystem2/6(i_in)
  Subsystem1/7(c_out) -> Subsystem2/7(c_in)
  Subsystem1/8(r_out) -> Subsystem2/8(r_in)
  Subsystem1/9(r_leak_out) -> Subsystem2/9(r_leak_in)
  Subsystem1/10(l_out) -> Subsystem2/10(l_in)
  Subsystem2/1(v_r_out) -> Subsystem3/1(v_r_in)
  Subsystem2/2(v_cap_out) -> Subsystem3/2(v_cap_in)
  Subsystem2/3(i_leak_out) -> Subsystem3/3(i_leak_in)
  Subsystem2/4(p_chg_out) -> Subsystem3/4(p_chg_in)
  Subsystem2/5(p_leak_out) -> Subsystem3/5(p_leak_in)
  Subsystem2/6(i_out) -> Subsystem3/6(i_in)
  Subsystem2/7(c_out) -> Subsystem3/7(c_in)
  Subsystem2/8(r_out) -> Subsystem3/8(r_in)
  Subsystem2/9(r_leak_out) -> Subsystem3/9(r_leak_in)
  Subsystem2/10(l_out) -> Subsystem3/10(l_in)
  Subsystem3/1(v_r_out) -> Out1/1
  Subsystem3/2(v_cap_out) -> Out2/1
  Subsystem3/3(i_leak_out) -> Out3/1
  Subsystem3/4(p_chg_out) -> Out4/1
  Subsystem3/5(p_leak_out) -> Out5/1
  Subsystem3/6(i_out) -> Out6/1
  Subsystem3/7(c_out) -> Out7/1
  Subsystem3/8(r_out) -> Out8/1
  Subsystem3/9(r_leak_out) -> Out9/1
  Subsystem3/10(l_out) -> Out10/1
  connections:
  Subsystem5/LConn1 -- Conn1/RConn1
  Subsystem5/LConn2 -- Conn3/RConn1
  Subsystem5/RConn1 -- Subsystem1/LConn1
  Subsystem5/RConn2 -- Subsystem1/LConn2
  Subsystem1/RConn1 -- Subsystem2/LConn1
  Subsystem1/RConn2 -- Subsystem2/LConn2
  Subsystem2/RConn1 -- Subsystem3/LConn1
  Subsystem2/RConn2 -- Subsystem3/LConn2
  Subsystem3/RConn1 -- Conn2/RConn1
  Subsystem3/RConn2 -- Conn4/RConn1

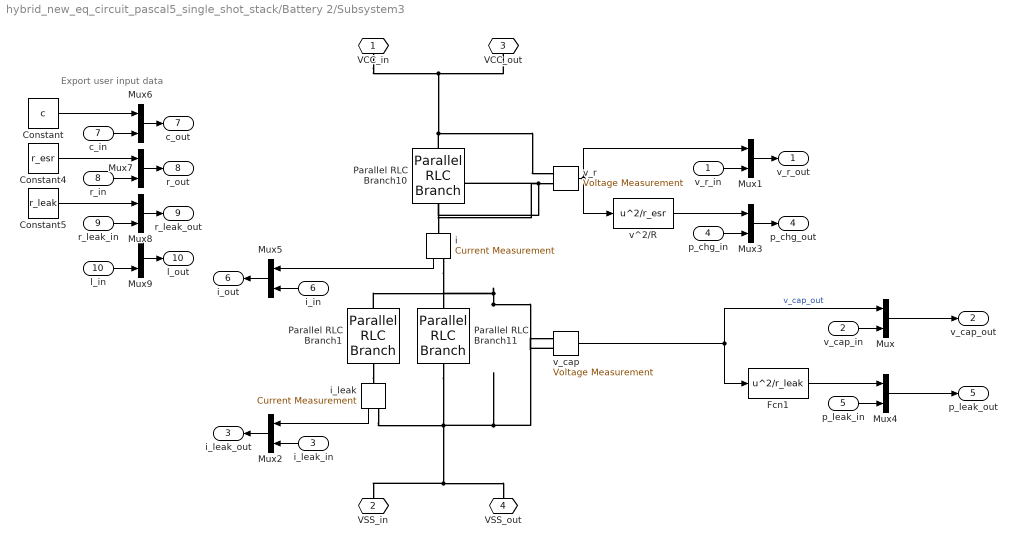
== system hybrid_new_eq_circuit_pascal5_single_shot_stack/Battery 2/Subsystem3 ==
  note: Export user input data
  v_r_in : Inport
  v_cap_in : Inport  Port=2
  i_leak_in : Inport  Port=3
  p_chg_in : Inport  Port=4
  p_leak_in : Inport  Port=5
  i_in : Inport  Port=6
  c_in : Inport  Port=7
  r_in : Inport  Port=8
  r_leak_in : Inport  Port=9
  l_in : Inport  Port=10
  Constant : Constant  Value=c
  Constant4 : Constant  Value=r_esr
  Constant5 : Constant  Value=r_leak
  Fcn1 : Fcn  Expr=u^2/r_leak
  Mux{,1..9} (10 alike) : Mux  Inputs=2
  Parallel RLC Branch1 : powerlib/Elements/Parallel RLC Branch  LConnTagsString=a  RConnTagsString=__new0  BranchType=R  Resistance=r_esr  Inductance=1e-3  SetiL0=off  InitialCurrent=0  Capacitance=1e-6  Setx0=off  InitialVoltage=0  Measurements=None
      settings: SourceProductName=Simscape Electrical
  Parallel RLC Branch10 : powerlib/Elements/Parallel RLC Branch  LConnTagsString=a  RConnTagsString=__new0  BranchType=R  Resistance=0.000001  Inductance=1e-3  SetiL0=off  InitialCurrent=0  Capacitance=1e-6  Setx0=off  InitialVoltage=0  Measurements=None
      settings: SourceProductName=Simscape Electrical
  Parallel RLC Branch11 : powerlib/Elements/Parallel RLC Branch  LConnTagsString=a  RConnTagsString=__new0  BranchType=C  Resistance=1  Inductance=1e-3  SetiL0=off  InitialCurrent=0  Capacitance=c  Setx0=on  InitialVoltage=v_init  Measurements=None
      settings: SourceProductName=Simscape Electrical
  i : powerlib/Measurements/Current Measurement  PhasorSimulation=off  OutputType=Complex  PSBequivalent=0
      settings: SourceProductName=Simscape Electrical
  i_leak : powerlib/Measurements/Current Measurement  PhasorSimulation=off  OutputType=Complex  PSBequivalent=0
      settings: SourceProductName=Simscape Electrical
  v^2/R : Fcn  Expr=u^2/r_esr
  v_cap : powerlib/Measurements/Voltage Measurement  PhasorSimulation=off  OutputType=Magnitude  PSBequivalent=0
      settings: SourceProductName=Simscape Electrical
  v_r : powerlib/Measurements/Voltage Measurement  PhasorSimulation=off  OutputType=Complex  PSBequivalent=0
      settings: SourceProductName=Simscape Electrical
  VCC_in : PMIOPort  Side=Left
  VSS_in : PMIOPort  Port=2  Side=Left
  VCC_out : PMIOPort  Tag=PMCPort  Port=3  Side=Right
  VSS_out : PMIOPort  Tag=PMCPort  Port=4  Side=Right
  v_r_out : Outport
  v_cap_out : Outport  Port=2
  i_leak_out : Outport  Port=3
  p_chg_out : Outport  Port=4
  p_leak_out : Outport  Port=5
  i_out : Outport  Port=6
  c_out : Outport  Port=7
  r_out : Outport  Port=8
  r_leak_out : Outport  Port=9
  l_out : Outport  Port=10
  wires:
  i_leak/1 -> Mux2/1
  v_r/1 -> Mux1/1, v^2/R/1
  Mux6/1 -> c_out/1
  Mux7/1 -> r_out/1
  Mux8/1 -> r_leak_out/1
  Mux9/1 -> l_out/1
  Constant/1 -> Mux6/1
  Constant4/1 -> Mux7/1
  Constant5/1 -> Mux8/1
  ? -> Mux9/1
  c_in/1 -> Mux6/2
  l_in/1 -> Mux9/2
  r_leak_in/1 -> Mux8/2
  r_in/1 -> Mux7/2
  p_chg_in/1 -> Mux3/2
  Mux3/1 -> p_chg_out/1
  v_r_in/1 -> Mux1/2
  Mux1/1 -> v_r_out/1
  v^2/R/1 -> Mux3/1
  Mux2/1 -> i_leak_out/1
  i_leak_in/1 -> Mux2/2
  i/1 -> Mux5/1
  Mux5/1 -> i_out/1
  i_in/1 -> Mux5/2
  p_leak_in/1 -> Mux4/2
  Mux4/1 -> p_leak_out/1
  Mux/1 -> v_cap_out/1
  v_cap_in/1 -> Mux/2
  Fcn1/1 -> Mux4/1
  v_cap/1 -> Fcn1/1, Mux/1  "v_cap_out"
  connections:
  VCC_in/RConn1 -- VCC_out/RConn1 -- v_r/LConn1 -- Parallel RLC Branch10/LConn1
  Parallel RLC Branch1/RConn1 -- i_leak/LConn1
  VSS_out/RConn1 -- VSS_in/RConn1 -- i_leak/RConn1 -- Parallel RLC Branch11/RConn1 -- v_cap/LConn2
  Parallel RLC Branch1/LConn1 -- i/RConn1 -- Parallel RLC Branch11/LConn1 -- v_cap/LConn1
  v_r/LConn2 -- Parallel RLC Branch10/RConn1 -- i/LConn1

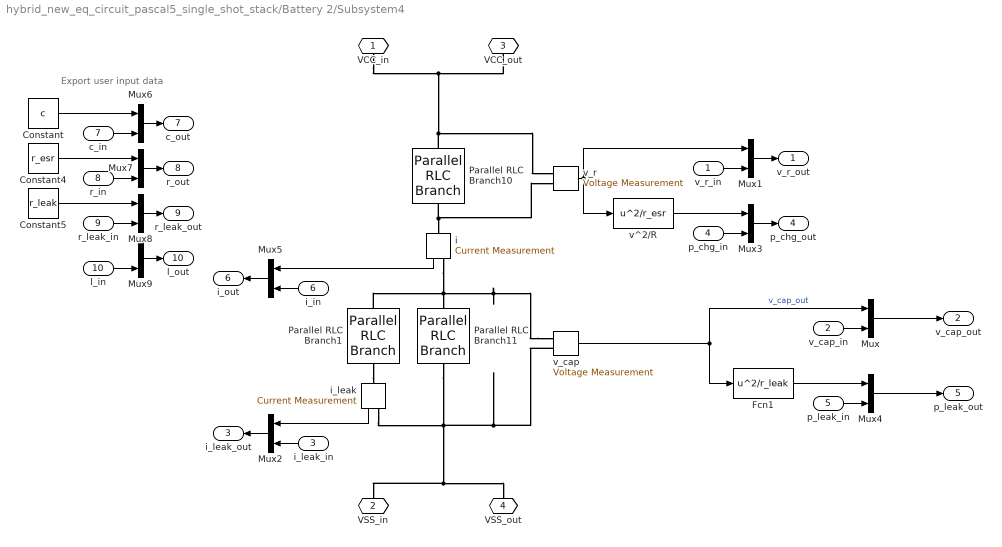
== system hybrid_new_eq_circuit_pascal5_single_shot_stack/Battery 2/Subsystem4 ==
  note: Export user input data
  v_r_in : Inport
  v_cap_in : Inport  Port=2
  i_leak_in : Inport  Port=3
  p_chg_in : Inport  Port=4
  p_leak_in : Inport  Port=5
  i_in : Inport  Port=6
  c_in : Inport  Port=7
  r_in : Inport  Port=8
  r_leak_in : Inport  Port=9
  l_in : Inport  Port=10
  Constant : Constant  Value=c
  Constant4 : Constant  Value=r_esr
  Constant5 : Constant  Value=r_leak
  Fcn1 : Fcn  Expr=u^2/r_leak
  Mux{,1..9} (10 alike) : Mux  Inputs=2
  Parallel RLC Branch1 : powerlib/Elements/Parallel RLC Branch  LConnTagsString=a  RConnTagsString=__new0  BranchType=R  Resistance=r_esr  Inductance=1e-3  SetiL0=off  InitialCurrent=0  Capacitance=1e-6  Setx0=off  InitialVoltage=0  Measurements=None
      settings: SourceProductName=Simscape Electrical
  Parallel RLC Branch10 : powerlib/Elements/Parallel RLC Branch  LConnTagsString=a  RConnTagsString=__new0  BranchType=R  Resistance=0.000001  Inductance=1e-3  SetiL0=off  InitialCurrent=0  Capacitance=1e-6  Setx0=off  InitialVoltage=0  Measurements=None
      settings: SourceProductName=Simscape Electrical
  Parallel RLC Branch11 : powerlib/Elements/Parallel RLC Branch  LConnTagsString=a  RConnTagsString=__new0  BranchType=C  Resistance=1  Inductance=1e-3  SetiL0=off  InitialCurrent=0  Capacitance=c  Setx0=on  InitialVoltage=v_init  Measurements=None
      settings: SourceProductName=Simscape Electrical
  i : powerlib/Measurements/Current Measurement  PhasorSimulation=off  OutputType=Complex  PSBequivalent=0
      settings: SourceProductName=Simscape Electrical
  i_leak : powerlib/Measurements/Current Measurement  PhasorSimulation=off  OutputType=Complex  PSBequivalent=0
      settings: SourceProductName=Simscape Electrical
  v^2/R : Fcn  Expr=u^2/r_esr
  v_cap : powerlib/Measurements/Voltage Measurement  PhasorSimulation=off  OutputType=Magnitude  PSBequivalent=0
      settings: SourceProductName=Simscape Electrical
  v_r : powerlib/Measurements/Voltage Measurement  PhasorSimulation=off  OutputType=Complex  PSBequivalent=0
      settings: SourceProductName=Simscape Electrical
  VCC_in : PMIOPort  Side=Left
  VSS_in : PMIOPort  Port=2  Side=Left
  VCC_out : PMIOPort  Tag=PMCPort  Port=3  Side=Right
  VSS_out : PMIOPort  Tag=PMCPort  Port=4  Side=Right
  v_r_out : Outport
  v_cap_out : Outport  Port=2
  i_leak_out : Outport  Port=3
  p_chg_out : Outport  Port=4
  p_leak_out : Outport  Port=5
  i_out : Outport  Port=6
  c_out : Outport  Port=7
  r_out : Outport  Port=8
  r_leak_out : Outport  Port=9
  l_out : Outport  Port=10
  wires:
  Fcn1/1 -> Mux4/1
  v_cap_in/1 -> Mux/2
  Mux/1 -> v_cap_out/1
  Mux4/1 -> p_leak_out/1
  p_leak_in/1 -> Mux4/2
  i_in/1 -> Mux5/2
  Mux5/1 -> i_out/1
  i/1 -> Mux5/1
  i_leak_in/1 -> Mux2/2
  Mux2/1 -> i_leak_out/1
  v^2/R/1 -> Mux3/1
  Mux1/1 -> v_r_out/1
  v_r_in/1 -> Mux1/2
  Mux3/1 -> p_chg_out/1
  p_chg_in/1 -> Mux3/2
  r_in/1 -> Mux7/2
  r_leak_in/1 -> Mux8/2
  l_in/1 -> Mux9/2
  c_in/1 -> Mux6/2
  ? -> Mux9/1
  Constant5/1 -> Mux8/1
  Constant4/1 -> Mux7/1
  Constant/1 -> Mux6/1
  Mux9/1 -> l_out/1
  Mux8/1 -> r_leak_out/1
  Mux7/1 -> r_out/1
  Mux6/1 -> c_out/1
  v_r/1 -> v^2/R/1, Mux1/1
  i_leak/1 -> Mux2/1
  v_cap/1 -> Mux/1, Fcn1/1  "v_cap_out"
  connections:
  i/LConn1 -- Parallel RLC Branch10/RConn1 -- v_r/LConn2
  Parallel RLC Branch10/LConn1 -- VCC_in/RConn1 -- VCC_out/RConn1 -- v_r/LConn1
  v_cap/LConn1 -- Parallel RLC Branch11/LConn1 -- i/RConn1 -- Parallel RLC Branch1/LConn1
  v_cap/LConn2 -- Parallel RLC Branch11/RConn1 -- i_leak/RConn1 -- VSS_in/RConn1 -- VSS_out/RConn1
  Parallel RLC Branch1/RConn1 -- i_leak/LConn1

== system hybrid_new_eq_circuit_pascal5_single_shot_stack/Battery 2/Subsystem8 ==
  note: Export user input data
  Constant : Constant  Value=c
  Constant4 : Constant  Value=r_esr
  Constant5 : Constant  Value=r_leak
  Fcn1 : Fcn  Expr=u^2/r_leak
  Parallel RLC Branch1 : powerlib/Elements/Parallel RLC Branch  LConnTagsString=a  RConnTagsString=__new0  BranchType=R  Resistance=r_leak  Inductance=1e-3  SetiL0=off  InitialCurrent=0  Capacitance=1e-6  Setx0=off  InitialVoltage=0  Measurements=None
      settings: SourceProductName=Simscape Electrical
  Parallel RLC Branch10 : powerlib/Elements/Parallel RLC Branch  LConnTagsString=a  RConnTagsString=__new0  BranchType=R  Resistance=0.000001  Inductance=1e-3  SetiL0=off  InitialCurrent=0  Capacitance=1e-6  Setx0=off  InitialVoltage=0  Measurements=None
      settings: SourceProductName=Simscape Electrical
  Parallel RLC Branch11 : powerlib/Elements/Parallel RLC Branch  LConnTagsString=a  RConnTagsString=__new0  BranchType=C  Resistance=1  Inductance=1e-3  SetiL0=off  InitialCurrent=0  Capacitance=c  Setx0=on  InitialVoltage=v_init  Measurements=None
      settings: SourceProductName=Simscape Electrical
  i : powerlib/Measurements/Current Measurement  PhasorSimulation=off  OutputType=Complex  PSBequivalent=0
      settings: SourceProductName=Simscape Electrical
  i_leak : powerlib/Measurements/Current Measurement  PhasorSimulation=off  OutputType=Complex  PSBequivalent=0
      settings: SourceProductName=Simscape Electrical
  v^2/R : Fcn  Expr=u^2/r_esr
  v_cap : powerlib/Measurements/Voltage Measurement  PhasorSimulation=off  OutputType=Magnitude  PSBequivalent=0
      settings: SourceProductName=Simscape Electrical
  v_r : powerlib/Measurements/Voltage Measurement  PhasorSimulation=off  OutputType=Complex  PSBequivalent=0
      settings: SourceProductName=Simscape Electrical
  VCC_in : PMIOPort  Side=Left
  VSS_in : PMIOPort  Port=2  Side=Left
  VCC_out : PMIOPort  Tag=PMCPort  Port=3  Side=Right
  VSS_out : PMIOPort  Tag=PMCPort  Port=4  Side=Right
  v_r_out : Outport
  v_cap_out : Outport  Port=2
  i_leak_out : Outport  Port=3
  p_chg_out : Outport  Port=4
  p_leak_out : Outport  Port=5
  i_out : Outport  Port=6
  c_out : Outport  Port=7
  r_out : Outport  Port=8
  r_leak_out : Outport  Port=9
  l_out : Outport  Port=10
  wires:
  v^2/R/1 -> p_chg_out/1
  Fcn1/1 -> p_leak_out/1
  v_cap/1 -> Fcn1/1, v_cap_out/1  "v_cap_out"
  i/1 -> i_out/1
  ? -> l_out/1
  Constant5/1 -> r_leak_out/1
  Constant4/1 -> r_out/1
  Constant/1 -> c_out/1
  v_r/1 -> v^2/R/1, v_r_out/1
  i_leak/1 -> i_leak_out/1
  connections:
  v_r/LConn2 -- Parallel RLC Branch10/RConn1 -- i/LConn1
  Parallel RLC Branch1/RConn1 -- i_leak/LConn1
  Parallel RLC Branch10/LConn1 -- v_r/LConn1 -- VCC_out/RConn1 -- VCC_in/RConn1
  i/RConn1 -- Parallel RLC Branch1/LConn1 -- v_cap/LConn1 -- Parallel RLC Branch11/LConn1
  i_leak/RConn1 -- v_cap/LConn2 -- VSS_in/RConn1 -- VSS_out/RConn1 -- Parallel RLC Branch11/RConn1

== system hybrid_new_eq_circuit_pascal5_single_shot_stack/Battery 3/Bus Merge2 ==
  bus_1_in : Inport
  bus_2_in : Inport  Port=2
  Bus Creator : BusCreator  Inputs=11
  Bus Selector : BusSelector  OutputSignals=signal1,v_cap_out,signal3,signal4,signal5,signal6,signal7,signal8,signal9,signal10,signal11
  Bus Selector1 : BusSelector  OutputSignals=signal1,v_cap_out,signal3,signal4,signal5,signal6,signal7,signal8,signal9,signal10,signal11
  Mux{1..11} (11 alike) : Mux  Inputs=2
  bus_out : Outport
  wires:
  bus_1_in/1 -> Bus Selector/1
  bus_2_in/1 -> Bus Selector1/1
  Bus Creator/1 -> bus_out/1
  Bus Selector/1 -> Mux1/1  "<signal1>"
  Bus Selector1/2 -> Mux2/2  "<v_cap_out>"
  Bus Selector/3 -> Mux3/1  "<signal3>"
  Bus Selector1/4 -> Mux4/2  "<signal4>"
  Bus Selector/5 -> Mux5/1  "<signal5>"
  Bus Selector1/6 -> Mux6/1  "<signal6>"
  Bus Selector/7 -> Mux7/1  "<signal7>"
  Bus Selector1/8 -> Mux8/1  "<signal8>"
  Bus Selector1/10 -> Mux10/1  "<signal10>"
  Bus Selector/11 -> Mux11/1  "<signal11>"
  Bus Selector/9 -> Mux9/1  "<signal9>"
  Bus Selector/2 -> Mux2/1  "<v_cap_out>"
  Bus Selector/4 -> Mux4/1  "<signal4>"
  Bus Selector/6 -> Mux6/2  "<signal6>"
  Bus Selector/8 -> Mux8/2  "<signal8>"
  Bus Selector/10 -> Mux10/2  "<signal10>"
  Bus Selector1/1 -> Mux1/2  "<signal1>"
  Bus Selector1/3 -> Mux3/2  "<signal3>"
  Bus Selector1/5 -> Mux5/2  "<signal5>"
  Bus Selector1/7 -> Mux7/2  "<signal7>"
  Bus Selector1/9 -> Mux9/2  "<signal9>"
  Bus Selector1/11 -> Mux11/2  "<signal11>"
  Mux1/1 -> Bus Creator/1
  Mux3/1 -> Bus Creator/3
  Mux5/1 -> Bus Creator/5
  Mux7/1 -> Bus Creator/7
  Mux9/1 -> Bus Creator/9
  Mux11/1 -> Bus Creator/11
  Mux2/1 -> Bus Creator/2  "v_cap_out"
  Mux4/1 -> Bus Creator/4
  Mux6/1 -> Bus Creator/6
  Mux8/1 -> Bus Creator/8
  Mux10/1 -> Bus Creator/10

== system hybrid_new_eq_circuit_pascal5_single_shot_stack/Battery 3/Subsystem ==
  In1 : Inport
  In2 : Inport  Port=2
  In3 : Inport  Port=3
  In4 : Inport  Port=4
  In5 : Inport  Port=5
  In6 : Inport  Port=6
  In7 : Inport  Port=7
  In8 : Inport  Port=8
  In9 : Inport  Port=9
  In10 : Inport  Port=10
  Subsystem1 : Subsystem  mask{c=c(5), r_esr=r(5), r_leak=r_leak, v_init=v_init(5)}
      mask prompts: c "Capacitance /F"; r_esr "Series resistance /ohm"; r_leak "Leakage resistance /ohm (inf for disabled)"; v_init "Initial capacitor voltage"
  Subsystem2 : Subsystem  mask{c=c(6), r_esr=r(6), r_leak=r_leak, v_init=v_init(6)}
      mask prompts: c "Capacitance /F"; r_esr "Series resistance /ohm"; r_leak "Leakage resistance /ohm (inf for disabled)"; v_init "Initial capacitor voltage"
  Subsystem3 : Subsystem  mask{c=c(7), r_esr=r(7), r_leak=r_leak, v_init=v_init(7)}
      mask prompts: c "Capacitance /F"; r_esr "Series resistance /ohm"; r_leak "Leakage resistance /ohm (inf for disabled)"; v_init "Initial capacitor voltage"
  Subsystem5 : Subsystem  mask{c=c(4), r_esr=r(4), r_leak=r_leak, v_init=v_init(4)}
      mask prompts: c "Capacitance /F"; r_esr "Series resistance /ohm"; r_leak "Leakage resistance /ohm (inf for disabled)"; v_init "Initial capacitor voltage"
  Conn1 : PMIOPort  Side=Left
  Conn2 : PMIOPort  Port=2  Side=Right
  Conn3 : PMIOPort  Port=3  Side=Left
  Conn4 : PMIOPort  Port=4  Side=Right
  Out1 : Outport
  Out2 : Outport  Port=2
  Out3 : Outport  Port=3
  Out4 : Outport  Port=4
  Out5 : Outport  Port=5
  Out6 : Outport  Port=6
  Out7 : Outport  Port=7
  Out8 : Outport  Port=8
  Out9 : Outport  Port=9
  Out10 : Outport  Port=10
  wires:
  In2/1 -> Subsystem5/2(v_cap_in)
  In9/1 -> Subsystem5/9(r_leak_in)
  In6/1 -> Subsystem5/6(i_in)
  In5/1 -> Subsystem5/5(p_leak_in)
  In4/1 -> Subsystem5/4(p_chg_in)
  In7/1 -> Subsystem5/7(c_in)
  In1/1 -> Subsystem5/1(v_r_in)
  In10/1 -> Subsystem5/10(l_in)
  In3/1 -> Subsystem5/3(i_leak_in)
  In8/1 -> Subsystem5/8(r_in)
  Subsystem5/1(v_r_out) -> Subsystem1/1(v_r_in)
  Subsystem5/2(v_cap_out) -> Subsystem1/2(v_cap_in)
  Subsystem5/3(i_leak_out) -> Subsystem1/3(i_leak_in)
  Subsystem5/4(p_chg_out) -> Subsystem1/4(p_chg_in)
  Subsystem5/5(p_leak_out) -> Subsystem1/5(p_leak_in)
  Subsystem5/6(i_out) -> Subsystem1/6(i_in)
  Subsystem5/7(c_out) -> Subsystem1/7(c_in)
  Subsystem5/8(r_out) -> Subsystem1/8(r_in)
  Subsystem5/9(r_leak_out) -> Subsystem1/9(r_leak_in)
  Subsystem5/10(l_out) -> Subsystem1/10(l_in)
  Subsystem1/1(v_r_out) -> Subsystem2/1(v_r_in)
  Subsystem1/2(v_cap_out) -> Subsystem2/2(v_cap_in)
  Subsystem1/3(i_leak_out) -> Subsystem2/3(i_leak_in)
  Subsystem1/4(p_chg_out) -> Subsystem2/4(p_chg_in)
  Subsystem1/5(p_leak_out) -> Subsystem2/5(p_leak_in)
  Subsystem1/6(i_out) -> Subsystem2/6(i_in)
  Subsystem1/7(c_out) -> Subsystem2/7(c_in)
  Subsystem1/8(r_out) -> Subsystem2/8(r_in)
  Subsystem1/9(r_leak_out) -> Subsystem2/9(r_leak_in)
  Subsystem1/10(l_out) -> Subsystem2/10(l_in)
  Subsystem2/1(v_r_out) -> Subsystem3/1(v_r_in)
  Subsystem2/2(v_cap_out) -> Subsystem3/2(v_cap_in)
  Subsystem2/3(i_leak_out) -> Subsystem3/3(i_leak_in)
  Subsystem2/4(p_chg_out) -> Subsystem3/4(p_chg_in)
  Subsystem2/5(p_leak_out) -> Subsystem3/5(p_leak_in)
  Subsystem2/6(i_out) -> Subsystem3/6(i_in)
  Subsystem2/7(c_out) -> Subsystem3/7(c_in)
  Subsystem2/8(r_out) -> Subsystem3/8(r_in)
  Subsystem2/9(r_leak_out) -> Subsystem3/9(r_leak_in)
  Subsystem2/10(l_out) -> Subsystem3/10(l_in)
  Subsystem3/1(v_r_out) -> Out1/1
  Subsystem3/2(v_cap_out) -> Out2/1
  Subsystem3/3(i_leak_out) -> Out3/1
  Subsystem3/4(p_chg_out) -> Out4/1
  Subsystem3/5(p_leak_out) -> Out5/1
  Subsystem3/6(i_out) -> Out6/1
  Subsystem3/7(c_out) -> Out7/1
  Subsystem3/8(r_out) -> Out8/1
  Subsystem3/9(r_leak_out) -> Out9/1
  Subsystem3/10(l_out) -> Out10/1
  connections:
  Subsystem5/LConn1 -- Conn1/RConn1
  Subsystem5/LConn2 -- Conn3/RConn1
  Subsystem5/RConn1 -- Subsystem1/LConn1
  Subsystem5/RConn2 -- Subsystem1/LConn2
  Subsystem1/RConn1 -- Subsystem2/LConn1
  Subsystem1/RConn2 -- Subsystem2/LConn2
  Subsystem2/RConn1 -- Subsystem3/LConn1
  Subsystem2/RConn2 -- Subsystem3/LConn2
  Subsystem3/RConn1 -- Conn2/RConn1
  Subsystem3/RConn2 -- Conn4/RConn1
